simulink model "Ex1_series_connection"  (R2024b)
settings: Solver=VariableStepAuto  StartTime=0.0  StopTime=3600  RelTol=1e-3
undefined symbols (not defined in the file): Ion, Lithium
libraries: spsBatteryLib x3, spsVoltageMeasurementLib x1, spspowerguiLib x1
settings Model: Creator=balaj  LastModifiedBy=balaj

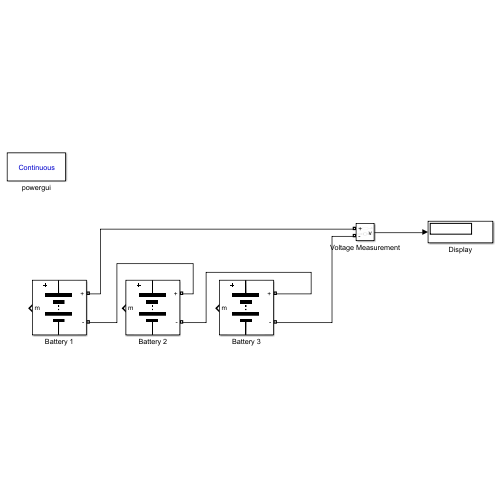
[thumbnail: Simulink's stored preview of the top-level diagram]
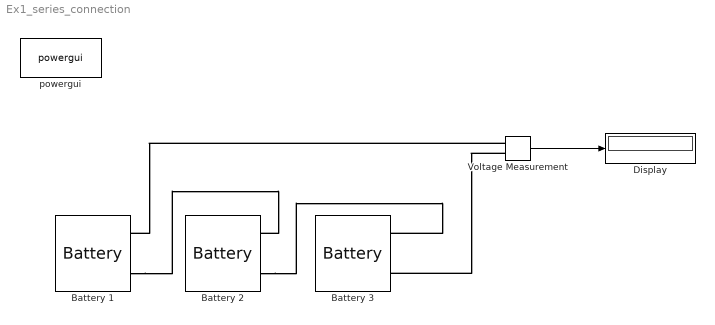
== system Ex1_series_connection ==
  Battery 1 : spsBatteryLib/Battery  BatType=Lithium-Ion  NomV=3.2  NomQ=5.4  SOC=100  Batt_Tr=30  PresetModel=off  MaxQ=5.4  MinV=2.775  FullV=3.7  Dis_rate=2.3478  R=0.0068519  Normal_OP=4.8835  expZone="[3.2974      0.2653]"
  Battery 2 : spsBatteryLib/Battery  BatType=Lithium-Ion  NomV=3.2  NomQ=5.4  SOC=100  Batt_Tr=30  PresetModel=off  MaxQ=5.4  MinV=2.775  FullV=3.7  Dis_rate=2.3478  R=0.0068519  Normal_OP=4.8835  expZone="[3.2974      0.2653]"
  Battery 3 : spsBatteryLib/Battery  BatType=Lithium-Ion  NomV=3.2  NomQ=5.4  SOC=100  Batt_Tr=30  PresetModel=off  MaxQ=5.4  MinV=2.775  FullV=3.7  Dis_rate=2.3478  R=0.0068519  Normal_OP=4.8835  expZone="[3.2974      0.2653]"
  Display : Display
  Voltage Measurement : spsVoltageMeasurementLib/Voltage Measurement  PhasorSimulation=off  OutputType=Complex  PSBequivalent=0
  powergui : spspowerguiLib/powergui  Priority=1  SimulationMode=Continuous  SampleTime=50e-6  frequency=60  Iterations=50  frequencyindice=0  Pbase=100e6  ErrMax=1e-4  UnitsV=kV  UnitsW=MW  buscounter=0  FunctionMessages=off  echomessages=off  EnableUseOfTLC=off  CurrentSourceSwitches=off  DisableSnubberDevices=off  DisableRonSwitches=off  DisableVfSwitches=off  DisplayEquations=off  AutomaticDiscreteSolvers=off  SolverType=Tustin/Backward Euler (TBE)  Interpol=off  ExternalGateDelay=off  methode=off  Ts=100  x0status=blocks  SPID=on  SwTol=0  HookPort=off  NonlinearTolerance=1e-4  nMaxIteration=100  ContinueOnMaxIteration=off  RestoreLinks=warning  ResistiveCurrentMeasurement=off  Frange=[0:2:500]  Ylog=off  Xlog=on  ShowGrid=off  save=off  variable=ZData  structure=0  ZoomFFT=off  StartTime=0.0  cycles=1  DisplayStyle=1  fundamental=60  FreqAxis=off  MaxFrequency=1000  frequencyindicesteady=1  RmsSteady=1  display=off
  wires:
  Voltage Measurement/1 -> Display/1
  connections:
  Battery 1/LConn2 -- Battery 2/LConn1
  Voltage Measurement/LConn1 -- Battery 1/LConn1
  Battery 2/LConn2 -- Battery 3/LConn1
  Voltage Measurement/LConn2 -- Battery 3/LConn2
